simulink model "msm_servo_loadest_ct"  (R2021b)
settings: Solver=daessc  StartTime=0.0  StopTime=simlength  RelTol=1e-3
undefined symbols (not defined in the file): Ale, Ble, Cle, K, Lle, load_torque, t_load
libraries: nesl_utility x5, fl_lib x3, mass_spring_mass_lib x1
settings Model: Creator=dbagn  LastModifiedBy=dbagn
settings SolverCC: AlgebraicLoopSolver=TrustRegion
settings DataIOCC: ReturnWorkspaceOutputs=off
settings DebuggingCC: SFMachineParentedDataDiag=warning

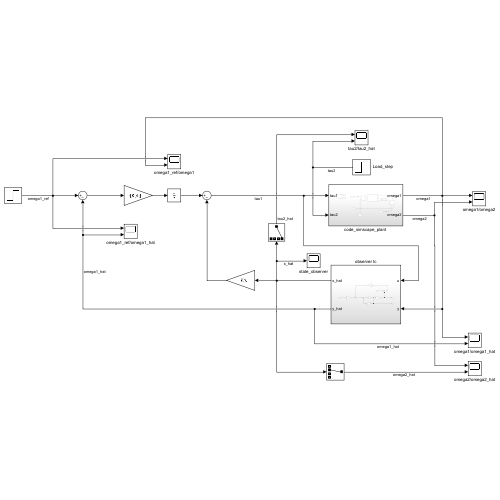
[thumbnail: Simulink's stored preview of the top-level diagram]
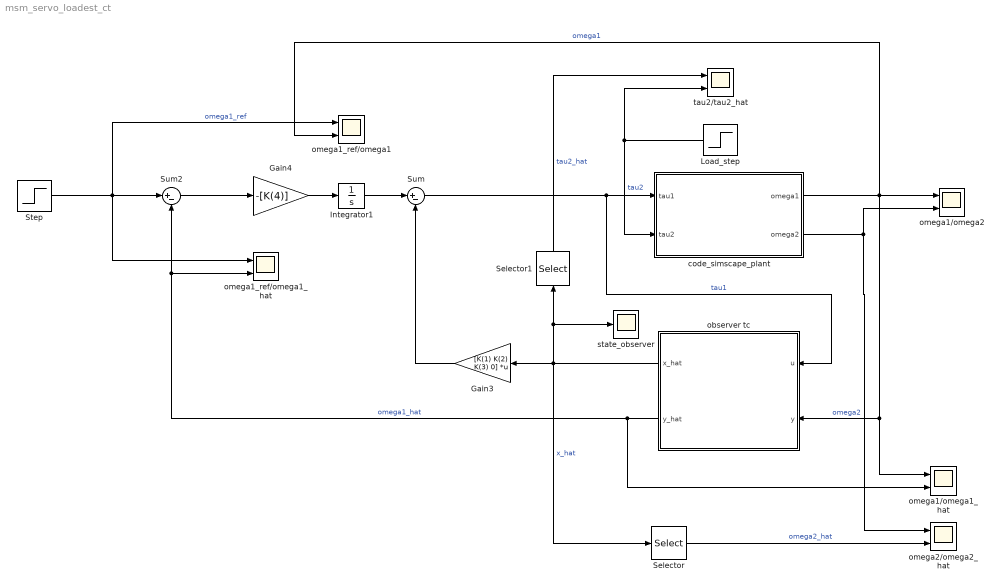
== system msm_servo_loadest_ct ==
  Gain3 : Gain  Gain=[K(1) K(2) K(3) 0]  Multiplication=Matrix(K*u)
  Gain4 : Gain  Gain=-[K(4)]
  Integrator1 : Integrator
  Load_step : Step  Time=t_load  After=load_torque  SampleTime=0
  Selector : Selector  InputPortWidth=4  IndexOptions=Index vector (dialog)  Indices=2  OutputSizes=1
  Selector1 : Selector  InputPortWidth=4  IndexOptions=Index vector (dialog)  Indices=4  OutputSizes=1
  Step : Step  SampleTime=0
  Sum : Sum  Inputs=|+-
  Sum2 : Sum  Inputs=|+-
  "code_simscape_plant " : Subsystem
  observer tc : Subsystem
  omega1/omega1_hat : Scope  NumInputPorts=2
  omega1/omega2 : Scope  NumInputPorts=2
  omega1_ref/omega1 : Scope  NumInputPorts=2
  omega1_ref/omega1_hat : Scope  NumInputPorts=2
  omega2/omega2_hat : Scope  NumInputPorts=2
  state_observer : Scope
  tau2/tau2_hat : Scope  NumInputPorts=2
  wires:
  Integrator1/1 -> Sum/1
  Gain4/1 -> Integrator1/1
  Step/1 -> omega1_ref/omega1/1, Sum2/1, omega1_ref/omega1_hat/1  "omega1_ref"
  Sum2/1 -> Gain4/1
  "code_simscape_plant "/1(omega1) -> omega1_ref/omega1/2, omega1/omega2/1, omega1/omega1_hat/1, observer tc/2(y)  "omega1"
  Sum/1 -> "code_simscape_plant "/1(tau1), observer tc/1(u)  "tau1"
  observer tc/1(x_hat) -> Selector/1, state_observer/1, Selector1/1, Gain3/1  "x_hat"
  "code_simscape_plant "/2(omega2) -> omega2/omega2_hat/1, omega1/omega2/2  "omega2"
  Load_step/1 -> tau2/tau2_hat/2, "code_simscape_plant "/2(tau2)  "tau2"
  observer tc/2(y_hat) -> omega1_ref/omega1_hat/2, Sum2/2, omega1/omega1_hat/2  "omega1_hat"
  Gain3/1 -> Sum/2
  Selector/1 -> omega2/omega2_hat/2  "omega2_hat"
  Selector1/1 -> tau2/tau2_hat/1  "tau2_hat"

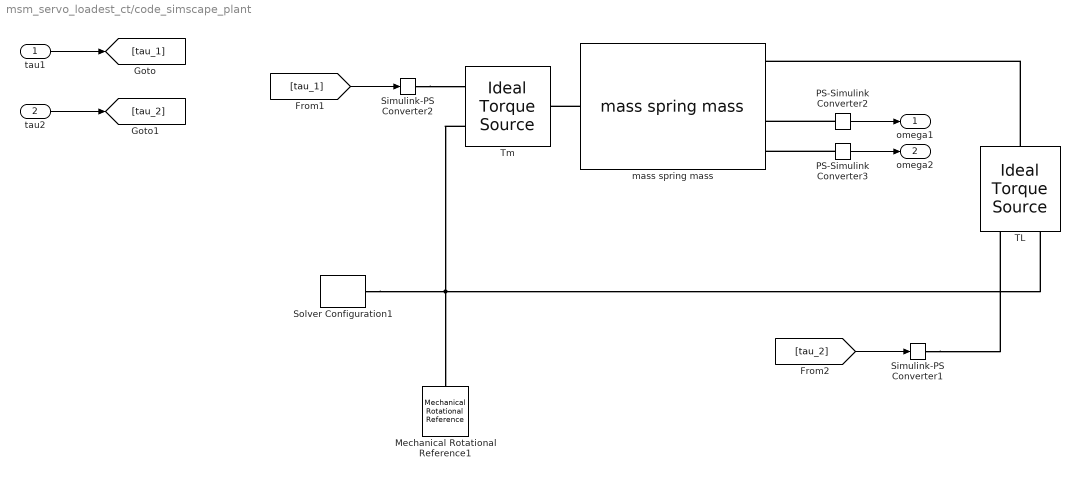
== system msm_servo_loadest_ct/code_simscape_plant  ==
  tau1 : Inport
  tau2 : Inport  Port=2
  Mechanical Rotational Reference1 : fl_lib/Mechanical/Rotational Elements/Mechanical Rotational Reference
  PS-Simulink Converter2 : nesl_utility/PS-Simulink Converter  PhysicalDomain=network_engine_domain  SubClassName=ps_output  LeftPortType=input  RightPortType=output  PseudoPeriodic=off  Frequencies=[]  Unit=1  AffineConversion=off
      settings: SourceProductBaseCode=PW,SS
  PS-Simulink Converter3 : nesl_utility/PS-Simulink Converter  PhysicalDomain=network_engine_domain  SubClassName=ps_output  LeftPortType=input  RightPortType=output  PseudoPeriodic=off  Frequencies=[]  Unit=1  AffineConversion=off
      settings: SourceProductBaseCode=PW,SS
  Simulink-PS Converter1 : nesl_utility/Simulink-PS Converter  PhysicalDomain=network_engine_domain  SubClassName=ps_input  LeftPortType=input  RightPortType=output  PseudoPeriodic=off  Frequencies=[]  NoiseDistribution=none  NoiseParameters=[]  Unit=1  AffineConversion=off  FilteringAndDerivatives=provide  SimscapeFilterOrder=1  InputFilterTimeConstant=0.001  UdotUserProvided=0
      settings: SourceProductBaseCode=PW,SS
  Simulink-PS Converter2 : nesl_utility/Simulink-PS Converter  PhysicalDomain=network_engine_domain  SubClassName=ps_input  LeftPortType=input  RightPortType=output  PseudoPeriodic=off  Frequencies=[]  NoiseDistribution=none  NoiseParameters=[]  Unit=1  AffineConversion=off  FilteringAndDerivatives=provide  SimscapeFilterOrder=1  InputFilterTimeConstant=0.001  UdotUserProvided=0
      settings: SourceProductBaseCode=PW,SS
  Solver Configuration1 : nesl_utility/Solver Configuration  PhysicalDomain=network_engine_domain  SubClassName=solver  LeftPortType=input  RightPortType=generic  Tones=[]  Harmonics=[]  SimulateNoise=off  Profile=off  UseLocalSampling=off  EnableSwitchedLinearOptims=on  FrequencyDomain=off  UseCCode=off  RelTol=0.001  AbsTol=1e-06  MinStep=1e-09  ToWorkspace=off  RevertToSquareIcSolve=off  NumHomotopyIterations=100  PhasorMode=off  PhasorModeNumHarmonics=1  DoDC=off  ResidualTolerance=1e-09  UseLocalSolver=off  LocalSolverChoice=NE_BACKWARD_EULER_ADVANCER  LocalSolverSampleTime=0.001  DoFixedCost=off  MaxNonlinIter=3  MaxModeIter=2  ComputeImpulses=off  ImpulseIterations=2  LinearAlgebra=auto  EquationFormulation=NE_TIME_EF  DelaysMemoryBudget=1024  AutomaticFiltering=on  FilteringTimeConstant=0.001  PartitionStorageMethod=AS_NEEDED  PartitionMemoryBudget=1024  PartitionMethod=ROBUST
      settings: SourceProductBaseCode=PW,SS
  TL : fl_lib/Mechanical/Mechanical Sources/Ideal Torque Source
  "Tm " : fl_lib/Mechanical/Mechanical Sources/Ideal Torque Source
  mass spring mass : mass_spring_mass_lib/mass spring mass  b1=b N*m/(rad/s)  J1=J1 kg*m^2  b2=b N*m/(rad/s)  J2=J2 kg*m^2  b_theta=b_theta N*m/(rad/s)  k_theta=k_theta N*m/rad  omega_1_specify=off  omega_1_priority=None  omega_1=0 rad/s  omega_1_nominal_specify=off  omega_1_nominal_unit=rad/s  omega_1_nominal_value=1  omega_2_specify=off  omega_2_priority=None  omega_2=0 rad/s  omega_2_nominal_specify=off  omega_2_nominal_unit=rad/s  omega_2_nominal_value=1  tau_1_specify=off  tau_1_priority=None  tau_1=0 N*m  tau_1_nominal_specify=off  tau_1_nominal_unit=N*m  tau_1_nominal_value=1  tau_2_specify=off  tau_2_priority=None  tau_2=0 N*m  tau_2_nominal_specify=off  tau_2_nominal_unit=N*m  tau_2_nominal_value=1  tau_theta_specify=off  tau_theta_priority=None  tau_theta=0 N*m  tau_theta_nominal_specify=off  tau_theta_nominal_unit=N*m  tau_theta_nominal_value=1
      settings: InternalSimscapePortConfiguration="{\"Bottom\":[],\"Left\":[{\"id\":\"S1\",\"label\":\"S1\",\"type\":\"foundation.mechanical.rotational.rotational\"}],\"Right\":[{\"id\":\"S2\",\"label\":\"S2\",\"type\":\"foundation.mechanical.rotational.rotational\"},{\"id\":\"tau_theta_out\",\"label\":\"tau_theta\",\"type\":\"output\"},{\"id\":\"omega1_out\",\"label\":\"omega1\",\"type\":\"output\"},{\"id\":\"omega2_out\",\"label\":\"omega2\",\"type\":\"output\"}],\"Top\":[]}"
  omega1 : Outport
  omega2 : Outport  Port=2
  wires:
  [tau_2] -> Simulink-PS Converter1/1
  tau2/1 -> [tau_2]
  [tau_1] -> Simulink-PS Converter2/1
  tau1/1 -> [tau_1]
  PS-Simulink Converter3/1 -> omega2/1
  PS-Simulink Converter2/1 -> omega1/1
  connections:
  Simulink-PS Converter2/RConn1 -- "Tm "/RConn1
  mass spring mass/LConn1 -- "Tm "/LConn1
  Simulink-PS Converter1/RConn1 -- TL/RConn1
  TL/LConn1 -- mass spring mass/RConn1
  PS-Simulink Converter3/LConn1 -- mass spring mass/RConn4
  PS-Simulink Converter2/LConn1 -- mass spring mass/RConn3
  Solver Configuration1/RConn1 -- "Tm "/RConn2 -- Mechanical Rotational Reference1/LConn1 -- TL/RConn2

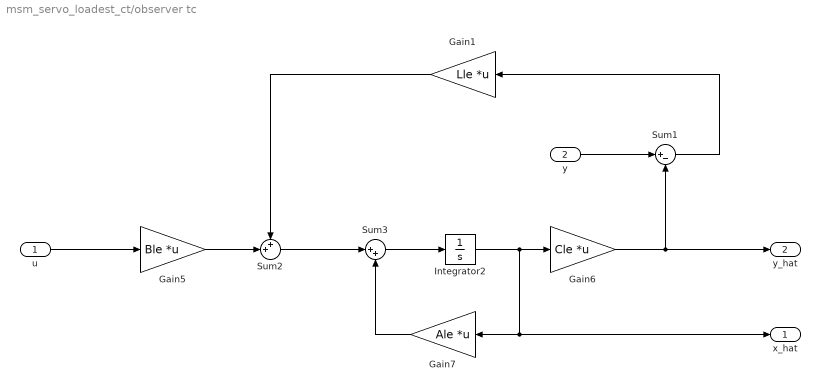
== system msm_servo_loadest_ct/observer tc ==
  u : Inport
  y : Inport  Port=2
  Gain1 : Gain  Gain=Lle  Multiplication=Matrix(K*u)
  Gain5 : Gain  Gain=Ble  Multiplication=Matrix(K*u)
  Gain6 : Gain  Gain=Cle  Multiplication=Matrix(K*u)
  Gain7 : Gain  Gain=Ale  Multiplication=Matrix(K*u)
  Integrator2 : Integrator
  Sum1 : Sum  Inputs=|+-
  Sum2 : Sum  Inputs=++|
  Sum3 : Sum  Inputs=|++
  x_hat : Outport
  y_hat : Outport  Port=2
  wires:
  Sum2/1 -> Sum3/1
  Integrator2/1 -> x_hat/1, Gain7/1, Gain6/1
  Sum3/1 -> Integrator2/1
  Gain7/1 -> Sum3/2
  y/1 -> Sum1/1
  Gain6/1 -> y_hat/1, Sum1/2
  Sum1/1 -> Gain1/1
  u/1 -> Gain5/1
  Gain1/1 -> Sum2/1
  Gain5/1 -> Sum2/2
